simulink model "sim_nomal_regulator"  (R2019a)
settings: Solver=FixedStepAuto  StartTime=0.0  StopTime=20  FixedStep=sT  RelTol=1e-3
InitFcn:
  | sim_param;
values from neighbouring files (symbols this model uses):
  bn = 50    [robot_param.m]    (also in sim_robot_param.m)
  bt = 50    [robot_param.m]    (also in sim_robot_param.m)
  foot_x = 0.07    [robot_param.m]    (also in sim_robot_param.m)
  foot_y = 0.045    [robot_param.m]    (also in sim_robot_param.m)
  foot_z = 0.01    [robot_param.m]    (also in sim_robot_param.m)
  height_plane = 0.025    [robot_param.m]    (also in sim_robot_param.m)
  inix = [0.00 0.00]'    [param.m]    (also in sim_param.m)
  iniXzmax = 0.05    [param.m]    (also in sim_param.m)
  iniXzmin = -0.05    [param.m]    (also in sim_param.m)
  iniy = [0.00 0.00]'    [param.m]    (also in sim_param.m)
  iniYzmax = 0.0625    [param.m]    (also in sim_param.m)
  iniYzmin = -0.0625    [param.m]    (also in sim_param.m)
  kn = 5000    [robot_param.m]    (also in sim_robot_param.m)
  kt = 5000    [robot_param.m]    (also in sim_robot_param.m)
  mu_d = 0.8    [robot_param.m]    (also in sim_robot_param.m)
  mu_s = 2    [robot_param.m]    (also in sim_robot_param.m)
  plane_x = 3    [robot_param.m]    (also in sim_robot_param.m = 6)
  plane_y = 1    [robot_param.m]    (also in sim_robot_param.m)
  R = 20    [param.m]    (also in sim_param.m = 1)
  sT = 0.02    [param.m]    (also in sim_param.m = 0.001)
  torso_offset_x = 0.0    (= 0)    [robot_param.m]    (also in sim_robot_param.m)
  torso_offset_z = -torso_z/2    (= -0.05)    [robot_param.m]    (also in sim_robot_param.m)
  torso_x = 0.1    [robot_param.m]    (also in sim_robot_param.m)
  torso_y = 0.08    [robot_param.m]    (also in sim_robot_param.m)
  torso_z = 0.10    (= 0.1)    [robot_param.m]    (also in sim_robot_param.m)
  w = sqrt(g/zc)    [param.m]    (also in sim_param.m)
  zvt = 1e-3    (= 0.001)    [robot_param.m]    (also in sim_robot_param.m)
undefined symbols (not defined in the file or in its folder): Ad, Bd, Cd, Dd, DiscIntNeverNeededParam, Discrete, sigbuilder_block, Time, X, Y, Z
libraries: nesl_utility x142, sm_lib x86, cstblocks x11, ctrlSharedLib x8
(part 3 of 6)

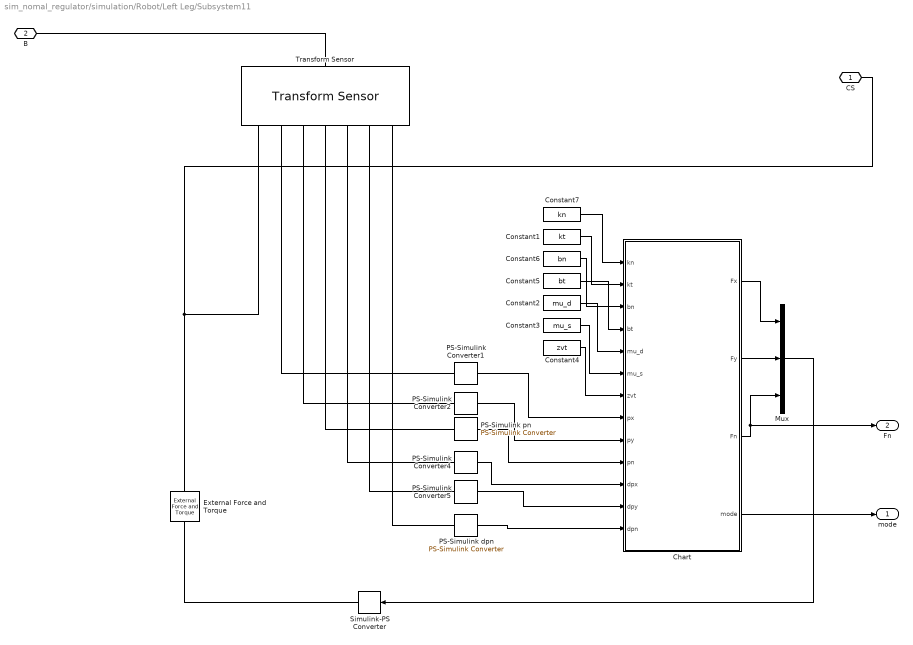
== system sim_nomal_regulator/simulation/Robot/Left Leg/Subsystem11 ==
  Chart : Stateflow chart  TreatAsAtomicUnit=on
  Constant1 : Constant  Value=kt
  Constant2 : Constant  Value=mu_d
  Constant3 : Constant  Value=mu_s
  Constant4 : Constant  Value=zvt
  Constant5 : Constant  Value=bt
  Constant6 : Constant  Value=bn
  Constant7 : Constant  Value=kn
  External Force and Torque : sm_lib/Forces and Torques/External Force and Torque  ForceResolutionFrame=AttachedFrame  EnableForceX=off  EnableForceY=off  EnableForceZ=off  EnableForce=on  TorqueResolutionFrame=AttachedFrame  EnableTorqueX=off  EnableTorqueY=off  EnableTorqueZ=off  EnableTorque=off
  Mux : Mux  Inputs=3
  PS-Simulink Converter1 : nesl_utility/PS-Simulink Converter  PhysicalDomain=network_engine_domain  SubClassName=ps_output  LeftPortType=input  RightPortType=output  PseudoPeriodic=off  Frequencies=[]  Unit=1  AffineConversion=off
  PS-Simulink Converter2 : nesl_utility/PS-Simulink Converter  PhysicalDomain=network_engine_domain  SubClassName=ps_output  LeftPortType=input  RightPortType=output  PseudoPeriodic=off  Frequencies=[]  Unit=1  AffineConversion=off
  PS-Simulink Converter4 : nesl_utility/PS-Simulink Converter  PhysicalDomain=network_engine_domain  SubClassName=ps_output  LeftPortType=input  RightPortType=output  PseudoPeriodic=off  Frequencies=[]  Unit=m/s  AffineConversion=off
  PS-Simulink Converter5 : nesl_utility/PS-Simulink Converter  PhysicalDomain=network_engine_domain  SubClassName=ps_output  LeftPortType=input  RightPortType=output  PseudoPeriodic=off  Frequencies=[]  Unit=m/s  AffineConversion=off
  PS-Simulink dpn : nesl_utility/PS-Simulink Converter  PhysicalDomain=network_engine_domain  SubClassName=ps_output  LeftPortType=input  RightPortType=output  PseudoPeriodic=off  Frequencies=[]  Unit=m/s  AffineConversion=off
  PS-Simulink pn : nesl_utility/PS-Simulink Converter  PhysicalDomain=network_engine_domain  SubClassName=ps_output  LeftPortType=input  RightPortType=output  PseudoPeriodic=off  Frequencies=[]  Unit=1  AffineConversion=off
  Simulink-PS Converter : nesl_utility/Simulink-PS Converter  PhysicalDomain=network_engine_domain  SubClassName=ps_input  LeftPortType=input  RightPortType=output  PseudoPeriodic=off  Frequencies=[]  NoiseDistribution=none  NoiseParameters=[]  Unit=N  AffineConversion=off  FilteringAndDerivatives=provide  SimscapeFilterOrder=1  InputFilterTimeConstant=0.001  UdotUserProvided=0
  Transform Sensor : sm_lib/Frames and Transforms/Transform Sensor  MeasurementFrame=World  SenseAngle=off  SenseAxis=off  SenseAngle1=off  SenseAngle2=off  SenseAngle3=off  SenseQ=off  SenseR=off  SenseOmegaX=off  SenseOmegaY=off  SenseOmegaZ=off  SenseOmega1=off  SenseOmega2=off  SenseOmega3=off  SenseQDot=off  SenseRDot=off  SenseAlphaX=off  SenseAlphaY=off  SenseAlphaZ=off  SenseAlpha1=off  SenseAlpha2=off  SenseAlpha3=off  SenseQDDot=off  SenseRDDot=off  SenseX=on  SenseY=on  SenseZ=on  SenseRad=off  SenseAzim=off  SenseDist=off  SenseInc=off  SenseXDot=on  SenseYDot=on  SenseZDot=on  SenseRadDot=off  SenseAzimDot=off  SenseDistDot=off  SenseIncDot=off  SenseXDDot=off  SenseYDDot=off  SenseZDDot=off  SenseRadDDot=off  SenseAzimDDot=off  SenseDistDDot=off  SenseIncDDot=off
  CS : PMIOPort  Side=Right
  B : PMIOPort  Port=2  Side=Left
  mode : Outport
  Fn : Outport  Port=2
  wires:
  PS-Simulink pn/1 -> Chart/10(pn)
  Constant5/1 -> Chart/4(bt)
  Constant3/1 -> Chart/6(mu_s)
  Constant6/1 -> Chart/3(bn)
  Constant4/1 -> Chart/7(zvt)
  Constant7/1 -> Chart/1(kn)
  PS-Simulink dpn/1 -> Chart/13(dpn)
  PS-Simulink Converter1/1 -> Chart/8(px)
  PS-Simulink Converter2/1 -> Chart/9(py)
  Constant1/1 -> Chart/2(kt)
  Constant2/1 -> Chart/5(mu_d)
  Chart/3(Fn) -> Mux/3, Fn/1
  Chart/2(Fy) -> Mux/2
  PS-Simulink Converter5/1 -> Chart/12(dpy)
  Chart/1(Fx) -> Mux/1
  PS-Simulink Converter4/1 -> Chart/11(dpx)
  Chart/4(mode) -> mode/1
  Mux/1 -> Simulink-PS Converter/1
  connections:
  Transform Sensor/RConn2 -- PS-Simulink Converter1/LConn1
  Transform Sensor/RConn5 -- PS-Simulink Converter4/LConn1
  Transform Sensor/RConn6 -- PS-Simulink Converter5/LConn1
  Transform Sensor/RConn7 -- PS-Simulink dpn/LConn1
  Transform Sensor/RConn4 -- PS-Simulink pn/LConn1
  Simulink-PS Converter/RConn1 -- External Force and Torque/LConn1
  Transform Sensor/RConn3 -- PS-Simulink Converter2/LConn1
  B/RConn1 -- Transform Sensor/LConn1
  External Force and Torque/RConn1 -- Transform Sensor/RConn1 -- CS/RConn1

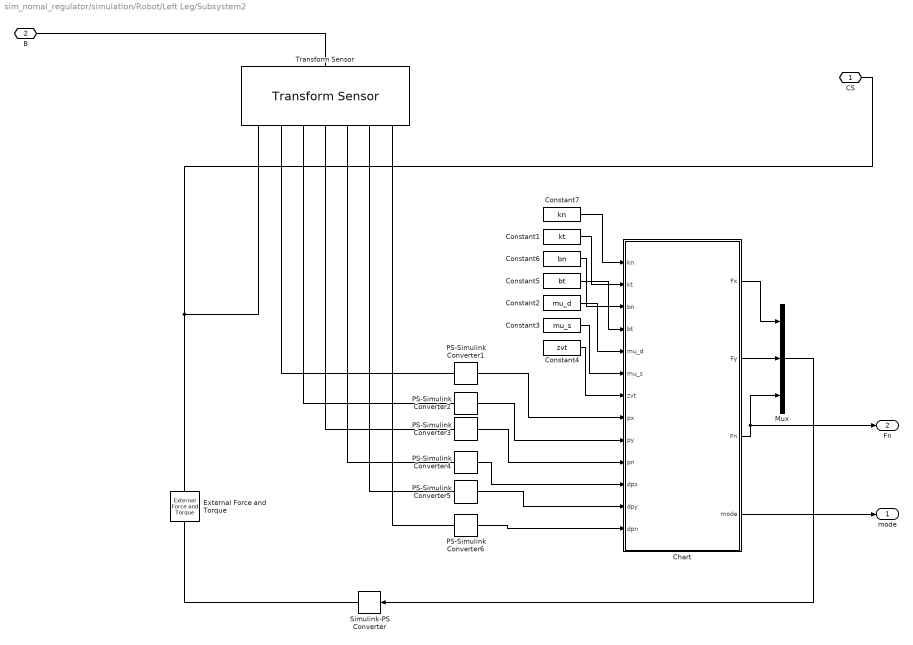
== system sim_nomal_regulator/simulation/Robot/Left Leg/Subsystem2 ==
  Chart : Stateflow chart  TreatAsAtomicUnit=on
  Constant1 : Constant  Value=kt
  Constant2 : Constant  Value=mu_d
  Constant3 : Constant  Value=mu_s
  Constant4 : Constant  Value=zvt
  Constant5 : Constant  Value=bt
  Constant6 : Constant  Value=bn
  Constant7 : Constant  Value=kn
  External Force and Torque : sm_lib/Forces and Torques/External Force and Torque  ForceResolutionFrame=AttachedFrame  EnableForceX=off  EnableForceY=off  EnableForceZ=off  EnableForce=on  TorqueResolutionFrame=AttachedFrame  EnableTorqueX=off  EnableTorqueY=off  EnableTorqueZ=off  EnableTorque=off
  Mux : Mux  Inputs=3
  PS-Simulink Converter1 : nesl_utility/PS-Simulink Converter  PhysicalDomain=network_engine_domain  SubClassName=ps_output  LeftPortType=input  RightPortType=output  PseudoPeriodic=off  Frequencies=[]  Unit=1  AffineConversion=off
  PS-Simulink Converter2 : nesl_utility/PS-Simulink Converter  PhysicalDomain=network_engine_domain  SubClassName=ps_output  LeftPortType=input  RightPortType=output  PseudoPeriodic=off  Frequencies=[]  Unit=1  AffineConversion=off
  PS-Simulink Converter3 : nesl_utility/PS-Simulink Converter  PhysicalDomain=network_engine_domain  SubClassName=ps_output  LeftPortType=input  RightPortType=output  PseudoPeriodic=off  Frequencies=[]  Unit=1  AffineConversion=off
  PS-Simulink Converter4 : nesl_utility/PS-Simulink Converter  PhysicalDomain=network_engine_domain  SubClassName=ps_output  LeftPortType=input  RightPortType=output  PseudoPeriodic=off  Frequencies=[]  Unit=m/s  AffineConversion=off
  PS-Simulink Converter5 : nesl_utility/PS-Simulink Converter  PhysicalDomain=network_engine_domain  SubClassName=ps_output  LeftPortType=input  RightPortType=output  PseudoPeriodic=off  Frequencies=[]  Unit=m/s  AffineConversion=off
  PS-Simulink Converter6 : nesl_utility/PS-Simulink Converter  PhysicalDomain=network_engine_domain  SubClassName=ps_output  LeftPortType=input  RightPortType=output  PseudoPeriodic=off  Frequencies=[]  Unit=m/s  AffineConversion=off
  Simulink-PS Converter : nesl_utility/Simulink-PS Converter  PhysicalDomain=network_engine_domain  SubClassName=ps_input  LeftPortType=input  RightPortType=output  PseudoPeriodic=off  Frequencies=[]  NoiseDistribution=none  NoiseParameters=[]  Unit=N  AffineConversion=off  FilteringAndDerivatives=provide  SimscapeFilterOrder=1  InputFilterTimeConstant=0.001  UdotUserProvided=0
  Transform Sensor : sm_lib/Frames and Transforms/Transform Sensor  MeasurementFrame=World  SenseAngle=off  SenseAxis=off  SenseAngle1=off  SenseAngle2=off  SenseAngle3=off  SenseQ=off  SenseR=off  SenseOmegaX=off  SenseOmegaY=off  SenseOmegaZ=off  SenseOmega1=off  SenseOmega2=off  SenseOmega3=off  SenseQDot=off  SenseRDot=off  SenseAlphaX=off  SenseAlphaY=off  SenseAlphaZ=off  SenseAlpha1=off  SenseAlpha2=off  SenseAlpha3=off  SenseQDDot=off  SenseRDDot=off  SenseX=on  SenseY=on  SenseZ=on  SenseRad=off  SenseAzim=off  SenseDist=off  SenseInc=off  SenseXDot=on  SenseYDot=on  SenseZDot=on  SenseRadDot=off  SenseAzimDot=off  SenseDistDot=off  SenseIncDot=off  SenseXDDot=off  SenseYDDot=off  SenseZDDot=off  SenseRadDDot=off  SenseAzimDDot=off  SenseDistDDot=off  SenseIncDDot=off
  CS : PMIOPort  Side=Right
  B : PMIOPort  Port=2  Side=Left
  mode : Outport
  Fn : Outport  Port=2
  wires:
  PS-Simulink Converter3/1 -> Chart/10(pn)
  Constant5/1 -> Chart/4(bt)
  Constant3/1 -> Chart/6(mu_s)
  Constant6/1 -> Chart/3(bn)
  Constant4/1 -> Chart/7(zvt)
  Constant7/1 -> Chart/1(kn)
  PS-Simulink Converter6/1 -> Chart/13(dpn)
  PS-Simulink Converter1/1 -> Chart/8(px)
  PS-Simulink Converter2/1 -> Chart/9(py)
  Constant1/1 -> Chart/2(kt)
  Constant2/1 -> Chart/5(mu_d)
  Chart/3(Fn) -> Fn/1, Mux/3
  Chart/2(Fy) -> Mux/2
  PS-Simulink Converter5/1 -> Chart/12(dpy)
  Chart/1(Fx) -> Mux/1
  PS-Simulink Converter4/1 -> Chart/11(dpx)
  Chart/4(mode) -> mode/1
  Mux/1 -> Simulink-PS Converter/1
  connections:
  Transform Sensor/RConn2 -- PS-Simulink Converter1/LConn1
  Transform Sensor/RConn5 -- PS-Simulink Converter4/LConn1
  Transform Sensor/RConn6 -- PS-Simulink Converter5/LConn1
  Transform Sensor/RConn7 -- PS-Simulink Converter6/LConn1
  Transform Sensor/RConn4 -- PS-Simulink Converter3/LConn1
  Simulink-PS Converter/RConn1 -- External Force and Torque/LConn1
  Transform Sensor/RConn3 -- PS-Simulink Converter2/LConn1
  B/RConn1 -- Transform Sensor/LConn1
  External Force and Torque/RConn1 -- Transform Sensor/RConn1 -- CS/RConn1

== system sim_nomal_regulator/simulation/Robot/Left Leg/Subsystem3 ==
  Chart : Stateflow chart  TreatAsAtomicUnit=on
  Constant1 : Constant  Value=kt
  Constant2 : Constant  Value=mu_d
  Constant3 : Constant  Value=mu_s
  Constant4 : Constant  Value=zvt
  Constant5 : Constant  Value=bt
  Constant6 : Constant  Value=bn
  Constant7 : Constant  Value=kn
  External Force and Torque : sm_lib/Forces and Torques/External Force and Torque  ForceResolutionFrame=AttachedFrame  EnableForceX=off  EnableForceY=off  EnableForceZ=off  EnableForce=on  TorqueResolutionFrame=AttachedFrame  EnableTorqueX=off  EnableTorqueY=off  EnableTorqueZ=off  EnableTorque=off
  Mux : Mux  Inputs=3
  PS-Simulink Converter1 : nesl_utility/PS-Simulink Converter  PhysicalDomain=network_engine_domain  SubClassName=ps_output  LeftPortType=input  RightPortType=output  PseudoPeriodic=off  Frequencies=[]  Unit=1  AffineConversion=off
  PS-Simulink Converter2 : nesl_utility/PS-Simulink Converter  PhysicalDomain=network_engine_domain  SubClassName=ps_output  LeftPortType=input  RightPortType=output  PseudoPeriodic=off  Frequencies=[]  Unit=1  AffineConversion=off
  PS-Simulink Converter3 : nesl_utility/PS-Simulink Converter  PhysicalDomain=network_engine_domain  SubClassName=ps_output  LeftPortType=input  RightPortType=output  PseudoPeriodic=off  Frequencies=[]  Unit=1  AffineConversion=off
  PS-Simulink Converter4 : nesl_utility/PS-Simulink Converter  PhysicalDomain=network_engine_domain  SubClassName=ps_output  LeftPortType=input  RightPortType=output  PseudoPeriodic=off  Frequencies=[]  Unit=m/s  AffineConversion=off
  PS-Simulink Converter5 : nesl_utility/PS-Simulink Converter  PhysicalDomain=network_engine_domain  SubClassName=ps_output  LeftPortType=input  RightPortType=output  PseudoPeriodic=off  Frequencies=[]  Unit=m/s  AffineConversion=off
  PS-Simulink Converter6 : nesl_utility/PS-Simulink Converter  PhysicalDomain=network_engine_domain  SubClassName=ps_output  LeftPortType=input  RightPortType=output  PseudoPeriodic=off  Frequencies=[]  Unit=m/s  AffineConversion=off
  Simulink-PS Converter : nesl_utility/Simulink-PS Converter  PhysicalDomain=network_engine_domain  SubClassName=ps_input  LeftPortType=input  RightPortType=output  PseudoPeriodic=off  Frequencies=[]  NoiseDistribution=none  NoiseParameters=[]  Unit=N  AffineConversion=off  FilteringAndDerivatives=provide  SimscapeFilterOrder=1  InputFilterTimeConstant=0.001  UdotUserProvided=0
  Transform Sensor : sm_lib/Frames and Transforms/Transform Sensor  MeasurementFrame=World  SenseAngle=off  SenseAxis=off  SenseAngle1=off  SenseAngle2=off  SenseAngle3=off  SenseQ=off  SenseR=off  SenseOmegaX=off  SenseOmegaY=off  SenseOmegaZ=off  SenseOmega1=off  SenseOmega2=off  SenseOmega3=off  SenseQDot=off  SenseRDot=off  SenseAlphaX=off  SenseAlphaY=off  SenseAlphaZ=off  SenseAlpha1=off  SenseAlpha2=off  SenseAlpha3=off  SenseQDDot=off  SenseRDDot=off  SenseX=on  SenseY=on  SenseZ=on  SenseRad=off  SenseAzim=off  SenseDist=off  SenseInc=off  SenseXDot=on  SenseYDot=on  SenseZDot=on  SenseRadDot=off  SenseAzimDot=off  SenseDistDot=off  SenseIncDot=off  SenseXDDot=off  SenseYDDot=off  SenseZDDot=off  SenseRadDDot=off  SenseAzimDDot=off  SenseDistDDot=off  SenseIncDDot=off
  CS : PMIOPort  Side=Right
  B : PMIOPort  Port=2  Side=Left
  mode : Outport
  Fn : Outport  Port=2
  wires:
  PS-Simulink Converter3/1 -> Chart/10(pn)
  Constant5/1 -> Chart/4(bt)
  Constant3/1 -> Chart/6(mu_s)
  Constant6/1 -> Chart/3(bn)
  Constant4/1 -> Chart/7(zvt)
  Constant7/1 -> Chart/1(kn)
  PS-Simulink Converter6/1 -> Chart/13(dpn)
  PS-Simulink Converter1/1 -> Chart/8(px)
  PS-Simulink Converter2/1 -> Chart/9(py)
  Constant1/1 -> Chart/2(kt)
  Constant2/1 -> Chart/5(mu_d)
  Chart/3(Fn) -> Fn/1, Mux/3
  Chart/2(Fy) -> Mux/2
  PS-Simulink Converter5/1 -> Chart/12(dpy)
  Chart/1(Fx) -> Mux/1
  PS-Simulink Converter4/1 -> Chart/11(dpx)
  Chart/4(mode) -> mode/1
  Mux/1 -> Simulink-PS Converter/1
  connections:
  Transform Sensor/RConn2 -- PS-Simulink Converter1/LConn1
  Transform Sensor/RConn5 -- PS-Simulink Converter4/LConn1
  Transform Sensor/RConn6 -- PS-Simulink Converter5/LConn1
  Transform Sensor/RConn7 -- PS-Simulink Converter6/LConn1
  Transform Sensor/RConn4 -- PS-Simulink Converter3/LConn1
  Simulink-PS Converter/RConn1 -- External Force and Torque/LConn1
  Transform Sensor/RConn3 -- PS-Simulink Converter2/LConn1
  B/RConn1 -- Transform Sensor/LConn1
  External Force and Torque/RConn1 -- Transform Sensor/RConn1 -- CS/RConn1

== system sim_nomal_regulator/simulation/Robot/Left Leg/Subsystem4 ==
  Chart : Stateflow chart  TreatAsAtomicUnit=on
  Constant1 : Constant  Value=kt
  Constant2 : Constant  Value=mu_d
  Constant3 : Constant  Value=mu_s
  Constant4 : Constant  Value=zvt
  Constant5 : Constant  Value=bt
  Constant6 : Constant  Value=bn
  Constant7 : Constant  Value=kn
  External Force and Torque : sm_lib/Forces and Torques/External Force and Torque  ForceResolutionFrame=AttachedFrame  EnableForceX=off  EnableForceY=off  EnableForceZ=off  EnableForce=on  TorqueResolutionFrame=AttachedFrame  EnableTorqueX=off  EnableTorqueY=off  EnableTorqueZ=off  EnableTorque=off
  Mux : Mux  Inputs=3
  PS-Simulink Converter1 : nesl_utility/PS-Simulink Converter  PhysicalDomain=network_engine_domain  SubClassName=ps_output  LeftPortType=input  RightPortType=output  PseudoPeriodic=off  Frequencies=[]  Unit=1  AffineConversion=off
  PS-Simulink Converter2 : nesl_utility/PS-Simulink Converter  PhysicalDomain=network_engine_domain  SubClassName=ps_output  LeftPortType=input  RightPortType=output  PseudoPeriodic=off  Frequencies=[]  Unit=1  AffineConversion=off
  PS-Simulink Converter4 : nesl_utility/PS-Simulink Converter  PhysicalDomain=network_engine_domain  SubClassName=ps_output  LeftPortType=input  RightPortType=output  PseudoPeriodic=off  Frequencies=[]  Unit=m/s  AffineConversion=off
  PS-Simulink Converter5 : nesl_utility/PS-Simulink Converter  PhysicalDomain=network_engine_domain  SubClassName=ps_output  LeftPortType=input  RightPortType=output  PseudoPeriodic=off  Frequencies=[]  Unit=m/s  AffineConversion=off
  PS-Simulink dpn : nesl_utility/PS-Simulink Converter  PhysicalDomain=network_engine_domain  SubClassName=ps_output  LeftPortType=input  RightPortType=output  PseudoPeriodic=off  Frequencies=[]  Unit=m/s  AffineConversion=off
  PS-Simulink pn : nesl_utility/PS-Simulink Converter  PhysicalDomain=network_engine_domain  SubClassName=ps_output  LeftPortType=input  RightPortType=output  PseudoPeriodic=off  Frequencies=[]  Unit=1  AffineConversion=off
  Simulink-PS Converter : nesl_utility/Simulink-PS Converter  PhysicalDomain=network_engine_domain  SubClassName=ps_input  LeftPortType=input  RightPortType=output  PseudoPeriodic=off  Frequencies=[]  NoiseDistribution=none  NoiseParameters=[]  Unit=N  AffineConversion=off  FilteringAndDerivatives=provide  SimscapeFilterOrder=1  InputFilterTimeConstant=0.001  UdotUserProvided=0
  Transform Sensor : sm_lib/Frames and Transforms/Transform Sensor  MeasurementFrame=World  SenseAngle=off  SenseAxis=off  SenseAngle1=off  SenseAngle2=off  SenseAngle3=off  SenseQ=off  SenseR=off  SenseOmegaX=off  SenseOmegaY=off  SenseOmegaZ=off  SenseOmega1=off  SenseOmega2=off  SenseOmega3=off  SenseQDot=off  SenseRDot=off  SenseAlphaX=off  SenseAlphaY=off  SenseAlphaZ=off  SenseAlpha1=off  SenseAlpha2=off  SenseAlpha3=off  SenseQDDot=off  SenseRDDot=off  SenseX=on  SenseY=on  SenseZ=on  SenseRad=off  SenseAzim=off  SenseDist=off  SenseInc=off  SenseXDot=on  SenseYDot=on  SenseZDot=on  SenseRadDot=off  SenseAzimDot=off  SenseDistDot=off  SenseIncDot=off  SenseXDDot=off  SenseYDDot=off  SenseZDDot=off  SenseRadDDot=off  SenseAzimDDot=off  SenseDistDDot=off  SenseIncDDot=off
  CS : PMIOPort  Side=Right
  B : PMIOPort  Port=2  Side=Left
  mode : Outport
  Fn : Outport  Port=2
  wires:
  PS-Simulink pn/1 -> Chart/10(pn)
  Constant5/1 -> Chart/4(bt)
  Constant3/1 -> Chart/6(mu_s)
  Constant6/1 -> Chart/3(bn)
  Constant4/1 -> Chart/7(zvt)
  Constant7/1 -> Chart/1(kn)
  PS-Simulink dpn/1 -> Chart/13(dpn)
  PS-Simulink Converter1/1 -> Chart/8(px)
  PS-Simulink Converter2/1 -> Chart/9(py)
  Constant1/1 -> Chart/2(kt)
  Constant2/1 -> Chart/5(mu_d)
  Chart/3(Fn) -> Mux/3, Fn/1
  Chart/2(Fy) -> Mux/2
  PS-Simulink Converter5/1 -> Chart/12(dpy)
  Chart/1(Fx) -> Mux/1
  PS-Simulink Converter4/1 -> Chart/11(dpx)
  Chart/4(mode) -> mode/1
  Mux/1 -> Simulink-PS Converter/1
  connections:
  Transform Sensor/RConn2 -- PS-Simulink Converter1/LConn1
  Transform Sensor/RConn5 -- PS-Simulink Converter4/LConn1
  Transform Sensor/RConn6 -- PS-Simulink Converter5/LConn1
  Transform Sensor/RConn7 -- PS-Simulink dpn/LConn1
  Transform Sensor/RConn4 -- PS-Simulink pn/LConn1
  Simulink-PS Converter/RConn1 -- External Force and Torque/LConn1
  Transform Sensor/RConn3 -- PS-Simulink Converter2/LConn1
  B/RConn1 -- Transform Sensor/LConn1
  External Force and Torque/RConn1 -- Transform Sensor/RConn1 -- CS/RConn1

== system sim_nomal_regulator/simulation/Robot/Left Leg/Subsystem5 ==
  Rigid Transform6 : sm_lib/Frames and Transforms/Rigid Transform  TranslationMethod=None  TranslationStandardOffset=0  TranslationLengthUnit=m  TranslationStandardAxis=+Z  TranslationCartesianOffset=[0 0 0]  TranslationROffset=0  TranslationROffsetUnits=m  TranslationZOffset=0  TranslationZOffsetUnits=m  TranslationThetaOffset=0  TranslationThetaOffsetUnits=deg  RotationMethod=StandardAxis  RotationAngleUnits=deg  RotationStandardAxis=+X  RotationAngle=-90  RotationArbitraryAxis=[0 0 1]  FollAlignAxisA=+X  BaseAlignAxisA=+Y  FollAlignAxisB=+Y  BaseAlignAxisB=+Z  RotationSequenceAxes=FollowerAxes  RotationSequence=XYX  RotationSequenceAngles=[0 0 0]  RotationSequenceAnglesUnits=deg  RotationMatrix=[1 0 0; 0 1 0; 0 0 1]
  Rigid Transform7 : sm_lib/Frames and Transforms/Rigid Transform  TranslationMethod=None  TranslationStandardOffset=0  TranslationLengthUnit=m  TranslationStandardAxis=+Z  TranslationCartesianOffset=[0 0 0]  TranslationROffset=0  TranslationROffsetUnits=m  TranslationZOffset=0  TranslationZOffsetUnits=m  TranslationThetaOffset=0  TranslationThetaOffsetUnits=deg  RotationMethod=StandardAxis  RotationAngleUnits=deg  RotationStandardAxis=+X  RotationAngle=90  RotationArbitraryAxis=[0 0 1]  FollAlignAxisA=+X  BaseAlignAxisA=+Y  FollAlignAxisB=+Y  BaseAlignAxisB=+Z  RotationSequenceAxes=FollowerAxes  RotationSequence=XYX  RotationSequenceAngles=[0 0 0]  RotationSequenceAnglesUnits=deg  RotationMatrix=[1 0 0; 0 1 0; 0 0 1]
  Y Revolute Joint2 : sm_lib/Joints/Revolute Joint  SenseConstraintForce=off  SenseConstraintForceX=off  SenseConstraintForceY=off  SenseConstraintForceZ=off  SenseConstraintTorque=off  SenseConstraintTorqueX=off  SenseConstraintTorqueY=off  SenseConstraintTorqueZ=off  SenseTotalForce=off  SenseTotalForceX=off  SenseTotalForceY=off  SenseTotalForceZ=off  SenseTotalTorque=off  SenseTotalTorqueX=off  SenseTotalTorqueY=off  SenseTotalTorqueZ=off  CompositeWrenchDir=FollowerOnBase  CompositeWrenchFrame=BaseFrame  EquilibriumPosition=0  EquilibriumPositionUnits=deg  SpringStiffness=joint_stiffness  SpringStiffnessUnits=N*m/rad  DampingCoefficient=joint_damping  DampingCoefficientUnits=N*m/(deg/s)  TorqueActuationMode=ComputedTorque  MotionActuationMode=InputMotion  SensePosition=off  SenseVelocity=off  SenseAcceleration=off  SenseTorqueForce=off  SenseLowerLimitTorqueForce=off  SenseUpperLimitTorqueForce=off  LowerLimitSpecify=off  LowerLimitBound=-90  LowerLimitBoundUnits=deg  LowerLimitStiffness=1e4  LowerLimitStiffnessUnits=N*m/deg  LowerLimitDamping=10  LowerLimitDampingUnits=N*m/(deg/s)  LowerLimitTransitionRegionWidth=0.1  LowerLimitTransitionRegionWidthUnits=deg  UpperLimitSpecify=off  UpperLimitBound=90  UpperLimitBoundUnits=deg  UpperLimitStiffness=1e4  UpperLimitStiffnessUnits=N*m/deg  UpperLimitDamping=10  UpperLimitDampingUnits=N*m/(deg/s)  UpperLimitTransitionRegionWidth=0.1  UpperLimitTransitionRegionWidthUnits=deg  PositionTargetSpecify=off  PositionTargetPriority=High  PositionTargetValue=0  PositionTargetValueUnits=deg  VelocityTargetSpecify=off  VelocityTargetPriority=High  VelocityTargetValue=0  VelocityTargetValueUnits=deg/s
  F : PMIOPort  Side=Right
  B : PMIOPort  Port=2  Side=Right
  qy : PMIOPort  Port=3  Side=Left
  connections:
  Rigid Transform7/LConn1 -- B/RConn1
  Rigid Transform6/RConn1 -- F/RConn1
  Y Revolute Joint2/LConn2 -- qy/RConn1
  Rigid Transform7/RConn1 -- Y Revolute Joint2/LConn1
  Rigid Transform6/LConn1 -- Y Revolute Joint2/RConn1

== system sim_nomal_regulator/simulation/Robot/Left Leg/Subsystem6 ==
  Rigid Transform : sm_lib/Frames and Transforms/Rigid Transform  TranslationMethod=None  TranslationStandardOffset=0  TranslationLengthUnit=m  TranslationStandardAxis=+Z  TranslationCartesianOffset=[0 0 0]  TranslationROffset=0  TranslationROffsetUnits=m  TranslationZOffset=0  TranslationZOffsetUnits=m  TranslationThetaOffset=0  TranslationThetaOffsetUnits=deg  RotationMethod=StandardAxis  RotationAngleUnits=deg  RotationStandardAxis=+Y  RotationAngle=90  RotationArbitraryAxis=[0 0 1]  FollAlignAxisA=+X  BaseAlignAxisA=+Y  FollAlignAxisB=+Y  BaseAlignAxisB=+Z  RotationSequenceAxes=FollowerAxes  RotationSequence=XYX  RotationSequenceAngles=[0 0 0]  RotationSequenceAnglesUnits=deg  RotationMatrix=[1 0 0; 0 1 0; 0 0 1]
  Rigid Transform1 : sm_lib/Frames and Transforms/Rigid Transform  TranslationMethod=None  TranslationStandardOffset=0  TranslationLengthUnit=m  TranslationStandardAxis=+Z  TranslationCartesianOffset=[0 0 0]  TranslationROffset=0  TranslationROffsetUnits=m  TranslationZOffset=0  TranslationZOffsetUnits=m  TranslationThetaOffset=0  TranslationThetaOffsetUnits=deg  RotationMethod=StandardAxis  RotationAngleUnits=deg  RotationStandardAxis=+Y  RotationAngle=-90  RotationArbitraryAxis=[0 0 1]  FollAlignAxisA=+X  BaseAlignAxisA=+Y  FollAlignAxisB=+Y  BaseAlignAxisB=+Z  RotationSequenceAxes=FollowerAxes  RotationSequence=XYX  RotationSequenceAngles=[0 0 0]  RotationSequenceAnglesUnits=deg  RotationMatrix=[1 0 0; 0 1 0; 0 0 1]
  Rigid Transform2 : sm_lib/Frames and Transforms/Rigid Transform  TranslationMethod=None  TranslationStandardOffset=0  TranslationLengthUnit=m  TranslationStandardAxis=+Z  TranslationCartesianOffset=[0 0 0]  TranslationROffset=0  TranslationROffsetUnits=m  TranslationZOffset=0  TranslationZOffsetUnits=m  TranslationThetaOffset=0  TranslationThetaOffsetUnits=deg  RotationMethod=StandardAxis  RotationAngleUnits=deg  RotationStandardAxis=+X  RotationAngle=-90  RotationArbitraryAxis=[0 0 1]  FollAlignAxisA=+X  BaseAlignAxisA=+Y  FollAlignAxisB=+Y  BaseAlignAxisB=+Z  RotationSequenceAxes=FollowerAxes  RotationSequence=XYX  RotationSequenceAngles=[0 0 0]  RotationSequenceAnglesUnits=deg  RotationMatrix=[1 0 0; 0 1 0; 0 0 1]
  Rigid Transform3 : sm_lib/Frames and Transforms/Rigid Transform  TranslationMethod=None  TranslationStandardOffset=0  TranslationLengthUnit=m  TranslationStandardAxis=+Z  TranslationCartesianOffset=[0 0 0]  TranslationROffset=0  TranslationROffsetUnits=m  TranslationZOffset=0  TranslationZOffsetUnits=m  TranslationThetaOffset=0  TranslationThetaOffsetUnits=deg  RotationMethod=StandardAxis  RotationAngleUnits=deg  RotationStandardAxis=+X  RotationAngle=90  RotationArbitraryAxis=[0 0 1]  FollAlignAxisA=+X  BaseAlignAxisA=+Y  FollAlignAxisB=+Y  BaseAlignAxisB=+Z  RotationSequenceAxes=FollowerAxes  RotationSequence=XYX  RotationSequenceAngles=[0 0 0]  RotationSequenceAnglesUnits=deg  RotationMatrix=[1 0 0; 0 1 0; 0 0 1]
  X Revolute Joint : sm_lib/Joints/Revolute Joint  SenseConstraintForce=off  SenseConstraintForceX=off  SenseConstraintForceY=off  SenseConstraintForceZ=off  SenseConstraintTorque=off  SenseConstraintTorqueX=off  SenseConstraintTorqueY=off  SenseConstraintTorqueZ=off  SenseTotalForce=off  SenseTotalForceX=off  SenseTotalForceY=off  SenseTotalForceZ=off  SenseTotalTorque=off  SenseTotalTorqueX=off  SenseTotalTorqueY=off  SenseTotalTorqueZ=off  CompositeWrenchDir=FollowerOnBase  CompositeWrenchFrame=BaseFrame  EquilibriumPosition=0  EquilibriumPositionUnits=deg  SpringStiffness=joint_stiffness  SpringStiffnessUnits=N*m/rad  DampingCoefficient=joint_damping  DampingCoefficientUnits=N*m/(deg/s)  TorqueActuationMode=ComputedTorque  MotionActuationMode=InputMotion  SensePosition=off  SenseVelocity=off  SenseAcceleration=off  SenseTorqueForce=off  SenseLowerLimitTorqueForce=off  SenseUpperLimitTorqueForce=off  LowerLimitSpecify=off  LowerLimitBound=-90  LowerLimitBoundUnits=deg  LowerLimitStiffness=1e4  LowerLimitStiffnessUnits=N*m/deg  LowerLimitDamping=10  LowerLimitDampingUnits=N*m/(deg/s)  LowerLimitTransitionRegionWidth=0.1  LowerLimitTransitionRegionWidthUnits=deg  UpperLimitSpecify=off  UpperLimitBound=90  UpperLimitBoundUnits=deg  UpperLimitStiffness=1e4  UpperLimitStiffnessUnits=N*m/deg  UpperLimitDamping=10  UpperLimitDampingUnits=N*m/(deg/s)  UpperLimitTransitionRegionWidth=0.1  UpperLimitTransitionRegionWidthUnits=deg  PositionTargetSpecify=off  PositionTargetPriority=High  PositionTargetValue=0  PositionTargetValueUnits=deg  VelocityTargetSpecify=off  VelocityTargetPriority=High  VelocityTargetValue=0  VelocityTargetValueUnits=deg/s
  Y Revolute Joint1 : sm_lib/Joints/Revolute Joint  SenseConstraintForce=off  SenseConstraintForceX=off  SenseConstraintForceY=off  SenseConstraintForceZ=off  SenseConstraintTorque=off  SenseConstraintTorqueX=off  SenseConstraintTorqueY=off  SenseConstraintTorqueZ=off  SenseTotalForce=off  SenseTotalForceX=off  SenseTotalForceY=off  SenseTotalForceZ=off  SenseTotalTorque=off  SenseTotalTorqueX=off  SenseTotalTorqueY=off  SenseTotalTorqueZ=off  CompositeWrenchDir=FollowerOnBase  CompositeWrenchFrame=BaseFrame  EquilibriumPosition=0  EquilibriumPositionUnits=deg  SpringStiffness=joint_stiffness  SpringStiffnessUnits=N*m/rad  DampingCoefficient=joint_damping  DampingCoefficientUnits=N*m/(deg/s)  TorqueActuationMode=ComputedTorque  MotionActuationMode=InputMotion  SensePosition=off  SenseVelocity=off  SenseAcceleration=off  SenseTorqueForce=off  SenseLowerLimitTorqueForce=off  SenseUpperLimitTorqueForce=off  LowerLimitSpecify=off  LowerLimitBound=-90  LowerLimitBoundUnits=deg  LowerLimitStiffness=1e4  LowerLimitStiffnessUnits=N*m/deg  LowerLimitDamping=10  LowerLimitDampingUnits=N*m/(deg/s)  LowerLimitTransitionRegionWidth=0.1  LowerLimitTransitionRegionWidthUnits=deg  UpperLimitSpecify=off  UpperLimitBound=90  UpperLimitBoundUnits=deg  UpperLimitStiffness=1e4  UpperLimitStiffnessUnits=N*m/deg  UpperLimitDamping=10  UpperLimitDampingUnits=N*m/(deg/s)  UpperLimitTransitionRegionWidth=0.1  UpperLimitTransitionRegionWidthUnits=deg  PositionTargetSpecify=off  PositionTargetPriority=High  PositionTargetValue=0  PositionTargetValueUnits=deg  VelocityTargetSpecify=off  VelocityTargetPriority=High  VelocityTargetValue=0  VelocityTargetValueUnits=deg/s
  F : PMIOPort  Side=Right
  B : PMIOPort  Port=2  Side=Right
  qx : PMIOPort  Port=3  Side=Left
  qy : PMIOPort  Port=4  Side=Left
  connections:
  Rigid Transform2/LConn1 -- Y Revolute Joint1/RConn1
  Rigid Transform/LConn1 -- X Revolute Joint/RConn1
  Rigid Transform1/LConn1 -- Rigid Transform2/RConn1
  Rigid Transform3/RConn1 -- Y Revolute Joint1/LConn1
  Rigid Transform1/RConn1 -- X Revolute Joint/LConn1
  Y Revolute Joint1/LConn2 -- qy/RConn1
  X Revolute Joint/LConn2 -- qx/RConn1
  Rigid Transform3/LConn1 -- B/RConn1
  Rigid Transform/RConn1 -- F/RConn1

== system sim_nomal_regulator/simulation/Robot/Left Leg/Subsystem7 ==
  Chart : Stateflow chart  TreatAsAtomicUnit=on
  Constant1 : Constant  Value=kt
  Constant2 : Constant  Value=mu_d
  Constant3 : Constant  Value=mu_s
  Constant4 : Constant  Value=zvt
  Constant5 : Constant  Value=bt
  Constant6 : Constant  Value=bn
  Constant7 : Constant  Value=kn
  External Force and Torque : sm_lib/Forces and Torques/External Force and Torque  ForceResolutionFrame=AttachedFrame  EnableForceX=off  EnableForceY=off  EnableForceZ=off  EnableForce=on  TorqueResolutionFrame=AttachedFrame  EnableTorqueX=off  EnableTorqueY=off  EnableTorqueZ=off  EnableTorque=off
  Mux : Mux  Inputs=3
  PS-Simulink Converter1 : nesl_utility/PS-Simulink Converter  PhysicalDomain=network_engine_domain  SubClassName=ps_output  LeftPortType=input  RightPortType=output  PseudoPeriodic=off  Frequencies=[]  Unit=1  AffineConversion=off
  PS-Simulink Converter2 : nesl_utility/PS-Simulink Converter  PhysicalDomain=network_engine_domain  SubClassName=ps_output  LeftPortType=input  RightPortType=output  PseudoPeriodic=off  Frequencies=[]  Unit=1  AffineConversion=off
  PS-Simulink Converter4 : nesl_utility/PS-Simulink Converter  PhysicalDomain=network_engine_domain  SubClassName=ps_output  LeftPortType=input  RightPortType=output  PseudoPeriodic=off  Frequencies=[]  Unit=m/s  AffineConversion=off
  PS-Simulink Converter5 : nesl_utility/PS-Simulink Converter  PhysicalDomain=network_engine_domain  SubClassName=ps_output  LeftPortType=input  RightPortType=output  PseudoPeriodic=off  Frequencies=[]  Unit=m/s  AffineConversion=off
  PS-Simulink dpn : nesl_utility/PS-Simulink Converter  PhysicalDomain=network_engine_domain  SubClassName=ps_output  LeftPortType=input  RightPortType=output  PseudoPeriodic=off  Frequencies=[]  Unit=m/s  AffineConversion=off
  PS-Simulink pn : nesl_utility/PS-Simulink Converter  PhysicalDomain=network_engine_domain  SubClassName=ps_output  LeftPortType=input  RightPortType=output  PseudoPeriodic=off  Frequencies=[]  Unit=1  AffineConversion=off
  Simulink-PS Converter : nesl_utility/Simulink-PS Converter  PhysicalDomain=network_engine_domain  SubClassName=ps_input  LeftPortType=input  RightPortType=output  PseudoPeriodic=off  Frequencies=[]  NoiseDistribution=none  NoiseParameters=[]  Unit=N  AffineConversion=off  FilteringAndDerivatives=provide  SimscapeFilterOrder=1  InputFilterTimeConstant=0.001  UdotUserProvided=0
  Transform Sensor : sm_lib/Frames and Transforms/Transform Sensor  MeasurementFrame=World  SenseAngle=off  SenseAxis=off  SenseAngle1=off  SenseAngle2=off  SenseAngle3=off  SenseQ=off  SenseR=off  SenseOmegaX=off  SenseOmegaY=off  SenseOmegaZ=off  SenseOmega1=off  SenseOmega2=off  SenseOmega3=off  SenseQDot=off  SenseRDot=off  SenseAlphaX=off  SenseAlphaY=off  SenseAlphaZ=off  SenseAlpha1=off  SenseAlpha2=off  SenseAlpha3=off  SenseQDDot=off  SenseRDDot=off  SenseX=on  SenseY=on  SenseZ=on  SenseRad=off  SenseAzim=off  SenseDist=off  SenseInc=off  SenseXDot=on  SenseYDot=on  SenseZDot=on  SenseRadDot=off  SenseAzimDot=off  SenseDistDot=off  SenseIncDot=off  SenseXDDot=off  SenseYDDot=off  SenseZDDot=off  SenseRadDDot=off  SenseAzimDDot=off  SenseDistDDot=off  SenseIncDDot=off
  CS : PMIOPort  Side=Right
  B : PMIOPort  Port=2  Side=Left
  mode : Outport
  Fn : Outport  Port=2
  wires:
  PS-Simulink pn/1 -> Chart/10(pn)
  Constant5/1 -> Chart/4(bt)
  Constant3/1 -> Chart/6(mu_s)
  Constant6/1 -> Chart/3(bn)
  Constant4/1 -> Chart/7(zvt)
  Constant7/1 -> Chart/1(kn)
  PS-Simulink dpn/1 -> Chart/13(dpn)
  PS-Simulink Converter1/1 -> Chart/8(px)
  PS-Simulink Converter2/1 -> Chart/9(py)
  Constant1/1 -> Chart/2(kt)
  Constant2/1 -> Chart/5(mu_d)
  Chart/3(Fn) -> Mux/3, Fn/1
  Chart/2(Fy) -> Mux/2
  PS-Simulink Converter5/1 -> Chart/12(dpy)
  Chart/1(Fx) -> Mux/1
  PS-Simulink Converter4/1 -> Chart/11(dpx)
  Chart/4(mode) -> mode/1
  Mux/1 -> Simulink-PS Converter/1
  connections:
  Transform Sensor/RConn2 -- PS-Simulink Converter1/LConn1
  Transform Sensor/RConn5 -- PS-Simulink Converter4/LConn1
  Transform Sensor/RConn6 -- PS-Simulink Converter5/LConn1
  Transform Sensor/RConn7 -- PS-Simulink dpn/LConn1
  Transform Sensor/RConn4 -- PS-Simulink pn/LConn1
  Simulink-PS Converter/RConn1 -- External Force and Torque/LConn1
  Transform Sensor/RConn3 -- PS-Simulink Converter2/LConn1
  B/RConn1 -- Transform Sensor/LConn1
  External Force and Torque/RConn1 -- Transform Sensor/RConn1 -- CS/RConn1

== system sim_nomal_regulator/simulation/Robot/Left Leg/Subsystem8 ==
  Chart : Stateflow chart  TreatAsAtomicUnit=on
  Constant1 : Constant  Value=kt
  Constant2 : Constant  Value=mu_d
  Constant3 : Constant  Value=mu_s
  Constant4 : Constant  Value=zvt
  Constant5 : Constant  Value=bt
  Constant6 : Constant  Value=bn
  Constant7 : Constant  Value=kn
  External Force and Torque : sm_lib/Forces and Torques/External Force and Torque  ForceResolutionFrame=AttachedFrame  EnableForceX=off  EnableForceY=off  EnableForceZ=off  EnableForce=on  TorqueResolutionFrame=AttachedFrame  EnableTorqueX=off  EnableTorqueY=off  EnableTorqueZ=off  EnableTorque=off
  Mux : Mux  Inputs=3
  PS-Simulink Converter1 : nesl_utility/PS-Simulink Converter  PhysicalDomain=network_engine_domain  SubClassName=ps_output  LeftPortType=input  RightPortType=output  PseudoPeriodic=off  Frequencies=[]  Unit=1  AffineConversion=off
  PS-Simulink Converter2 : nesl_utility/PS-Simulink Converter  PhysicalDomain=network_engine_domain  SubClassName=ps_output  LeftPortType=input  RightPortType=output  PseudoPeriodic=off  Frequencies=[]  Unit=1  AffineConversion=off
  PS-Simulink Converter4 : nesl_utility/PS-Simulink Converter  PhysicalDomain=network_engine_domain  SubClassName=ps_output  LeftPortType=input  RightPortType=output  PseudoPeriodic=off  Frequencies=[]  Unit=m/s  AffineConversion=off
  PS-Simulink Converter5 : nesl_utility/PS-Simulink Converter  PhysicalDomain=network_engine_domain  SubClassName=ps_output  LeftPortType=input  RightPortType=output  PseudoPeriodic=off  Frequencies=[]  Unit=m/s  AffineConversion=off
  PS-Simulink dpn : nesl_utility/PS-Simulink Converter  PhysicalDomain=network_engine_domain  SubClassName=ps_output  LeftPortType=input  RightPortType=output  PseudoPeriodic=off  Frequencies=[]  Unit=m/s  AffineConversion=off
  PS-Simulink pn : nesl_utility/PS-Simulink Converter  PhysicalDomain=network_engine_domain  SubClassName=ps_output  LeftPortType=input  RightPortType=output  PseudoPeriodic=off  Frequencies=[]  Unit=1  AffineConversion=off
  Simulink-PS Converter : nesl_utility/Simulink-PS Converter  PhysicalDomain=network_engine_domain  SubClassName=ps_input  LeftPortType=input  RightPortType=output  PseudoPeriodic=off  Frequencies=[]  NoiseDistribution=none  NoiseParameters=[]  Unit=N  AffineConversion=off  FilteringAndDerivatives=provide  SimscapeFilterOrder=1  InputFilterTimeConstant=0.001  UdotUserProvided=0
  Transform Sensor : sm_lib/Frames and Transforms/Transform Sensor  MeasurementFrame=World  SenseAngle=off  SenseAxis=off  SenseAngle1=off  SenseAngle2=off  SenseAngle3=off  SenseQ=off  SenseR=off  SenseOmegaX=off  SenseOmegaY=off  SenseOmegaZ=off  SenseOmega1=off  SenseOmega2=off  SenseOmega3=off  SenseQDot=off  SenseRDot=off  SenseAlphaX=off  SenseAlphaY=off  SenseAlphaZ=off  SenseAlpha1=off  SenseAlpha2=off  SenseAlpha3=off  SenseQDDot=off  SenseRDDot=off  SenseX=on  SenseY=on  SenseZ=on  SenseRad=off  SenseAzim=off  SenseDist=off  SenseInc=off  SenseXDot=on  SenseYDot=on  SenseZDot=on  SenseRadDot=off  SenseAzimDot=off  SenseDistDot=off  SenseIncDot=off  SenseXDDot=off  SenseYDDot=off  SenseZDDot=off  SenseRadDDot=off  SenseAzimDDot=off  SenseDistDDot=off  SenseIncDDot=off
  CS : PMIOPort  Side=Right
  B : PMIOPort  Port=2  Side=Left
  mode : Outport
  Fn : Outport  Port=2
  wires:
  PS-Simulink pn/1 -> Chart/10(pn)
  Constant5/1 -> Chart/4(bt)
  Constant3/1 -> Chart/6(mu_s)
  Constant6/1 -> Chart/3(bn)
  Constant4/1 -> Chart/7(zvt)
  Constant7/1 -> Chart/1(kn)
  PS-Simulink dpn/1 -> Chart/13(dpn)
  PS-Simulink Converter1/1 -> Chart/8(px)
  PS-Simulink Converter2/1 -> Chart/9(py)
  Constant1/1 -> Chart/2(kt)
  Constant2/1 -> Chart/5(mu_d)
  Chart/3(Fn) -> Mux/3, Fn/1
  Chart/2(Fy) -> Mux/2
  PS-Simulink Converter5/1 -> Chart/12(dpy)
  Chart/1(Fx) -> Mux/1
  PS-Simulink Converter4/1 -> Chart/11(dpx)
  Chart/4(mode) -> mode/1
  Mux/1 -> Simulink-PS Converter/1
  connections:
  Transform Sensor/RConn2 -- PS-Simulink Converter1/LConn1
  Transform Sensor/RConn5 -- PS-Simulink Converter4/LConn1
  Transform Sensor/RConn6 -- PS-Simulink Converter5/LConn1
  Transform Sensor/RConn7 -- PS-Simulink dpn/LConn1
  Transform Sensor/RConn4 -- PS-Simulink pn/LConn1
  Simulink-PS Converter/RConn1 -- External Force and Torque/LConn1
  Transform Sensor/RConn3 -- PS-Simulink Converter2/LConn1
  B/RConn1 -- Transform Sensor/LConn1
  External Force and Torque/RConn1 -- Transform Sensor/RConn1 -- CS/RConn1

== system sim_nomal_regulator/simulation/Robot/Left Leg/Subsystem9 ==
  Chart : Stateflow chart  TreatAsAtomicUnit=on
  Constant1 : Constant  Value=kt
  Constant2 : Constant  Value=mu_d
  Constant3 : Constant  Value=mu_s
  Constant4 : Constant  Value=zvt
  Constant5 : Constant  Value=bt
  Constant6 : Constant  Value=bn
  Constant7 : Constant  Value=kn
  External Force and Torque : sm_lib/Forces and Torques/External Force and Torque  ForceResolutionFrame=AttachedFrame  EnableForceX=off  EnableForceY=off  EnableForceZ=off  EnableForce=on  TorqueResolutionFrame=AttachedFrame  EnableTorqueX=off  EnableTorqueY=off  EnableTorqueZ=off  EnableTorque=off
  Mux : Mux  Inputs=3
  PS-Simulink Converter1 : nesl_utility/PS-Simulink Converter  PhysicalDomain=network_engine_domain  SubClassName=ps_output  LeftPortType=input  RightPortType=output  PseudoPeriodic=off  Frequencies=[]  Unit=1  AffineConversion=off
  PS-Simulink Converter2 : nesl_utility/PS-Simulink Converter  PhysicalDomain=network_engine_domain  SubClassName=ps_output  LeftPortType=input  RightPortType=output  PseudoPeriodic=off  Frequencies=[]  Unit=1  AffineConversion=off
  PS-Simulink Converter4 : nesl_utility/PS-Simulink Converter  PhysicalDomain=network_engine_domain  SubClassName=ps_output  LeftPortType=input  RightPortType=output  PseudoPeriodic=off  Frequencies=[]  Unit=m/s  AffineConversion=off
  PS-Simulink Converter5 : nesl_utility/PS-Simulink Converter  PhysicalDomain=network_engine_domain  SubClassName=ps_output  LeftPortType=input  RightPortType=output  PseudoPeriodic=off  Frequencies=[]  Unit=m/s  AffineConversion=off
  PS-Simulink dpn : nesl_utility/PS-Simulink Converter  PhysicalDomain=network_engine_domain  SubClassName=ps_output  LeftPortType=input  RightPortType=output  PseudoPeriodic=off  Frequencies=[]  Unit=m/s  AffineConversion=off
  PS-Simulink pn : nesl_utility/PS-Simulink Converter  PhysicalDomain=network_engine_domain  SubClassName=ps_output  LeftPortType=input  RightPortType=output  PseudoPeriodic=off  Frequencies=[]  Unit=1  AffineConversion=off
  Simulink-PS Converter : nesl_utility/Simulink-PS Converter  PhysicalDomain=network_engine_domain  SubClassName=ps_input  LeftPortType=input  RightPortType=output  PseudoPeriodic=off  Frequencies=[]  NoiseDistribution=none  NoiseParameters=[]  Unit=N  AffineConversion=off  FilteringAndDerivatives=provide  SimscapeFilterOrder=1  InputFilterTimeConstant=0.001  UdotUserProvided=0
  Transform Sensor : sm_lib/Frames and Transforms/Transform Sensor  MeasurementFrame=World  SenseAngle=off  SenseAxis=off  SenseAngle1=off  SenseAngle2=off  SenseAngle3=off  SenseQ=off  SenseR=off  SenseOmegaX=off  SenseOmegaY=off  SenseOmegaZ=off  SenseOmega1=off  SenseOmega2=off  SenseOmega3=off  SenseQDot=off  SenseRDot=off  SenseAlphaX=off  SenseAlphaY=off  SenseAlphaZ=off  SenseAlpha1=off  SenseAlpha2=off  SenseAlpha3=off  SenseQDDot=off  SenseRDDot=off  SenseX=on  SenseY=on  SenseZ=on  SenseRad=off  SenseAzim=off  SenseDist=off  SenseInc=off  SenseXDot=on  SenseYDot=on  SenseZDot=on  SenseRadDot=off  SenseAzimDot=off  SenseDistDot=off  SenseIncDot=off  SenseXDDot=off  SenseYDDot=off  SenseZDDot=off  SenseRadDDot=off  SenseAzimDDot=off  SenseDistDDot=off  SenseIncDDot=off
  CS : PMIOPort  Side=Right
  B : PMIOPort  Port=2  Side=Left
  mode : Outport
  Fn : Outport  Port=2
  wires:
  PS-Simulink pn/1 -> Chart/10(pn)
  Constant5/1 -> Chart/4(bt)
  Constant3/1 -> Chart/6(mu_s)
  Constant6/1 -> Chart/3(bn)
  Constant4/1 -> Chart/7(zvt)
  Constant7/1 -> Chart/1(kn)
  PS-Simulink dpn/1 -> Chart/13(dpn)
  PS-Simulink Converter1/1 -> Chart/8(px)
  PS-Simulink Converter2/1 -> Chart/9(py)
  Constant1/1 -> Chart/2(kt)
  Constant2/1 -> Chart/5(mu_d)
  Chart/3(Fn) -> Mux/3, Fn/1
  Chart/2(Fy) -> Mux/2
  PS-Simulink Converter5/1 -> Chart/12(dpy)
  Chart/1(Fx) -> Mux/1
  PS-Simulink Converter4/1 -> Chart/11(dpx)
  Chart/4(mode) -> mode/1
  Mux/1 -> Simulink-PS Converter/1
  connections:
  Transform Sensor/RConn2 -- PS-Simulink Converter1/LConn1
  Transform Sensor/RConn5 -- PS-Simulink Converter4/LConn1
  Transform Sensor/RConn6 -- PS-Simulink Converter5/LConn1
  Transform Sensor/RConn7 -- PS-Simulink dpn/LConn1
  Transform Sensor/RConn4 -- PS-Simulink pn/LConn1
  Simulink-PS Converter/RConn1 -- External Force and Torque/LConn1
  Transform Sensor/RConn3 -- PS-Simulink Converter2/LConn1
  B/RConn1 -- Transform Sensor/LConn1
  External Force and Torque/RConn1 -- Transform Sensor/RConn1 -- CS/RConn1
